simulink model "momentum_envelope_test"  (R2018b)
settings: Solver=ode4  StartTime=0.0  StopTime=500.0  FixedStep=0.1  MaxStep=1e-1  RelTol=1e-5  AbsTol=1e-5
undefined symbols (not defined in the file): DiscIntNeverNeededParam, fswParams
libraries: rwa_allocation_lib x1
settings Model: Creator=taylorreynolds  LastModifiedBy=taylorreynolds

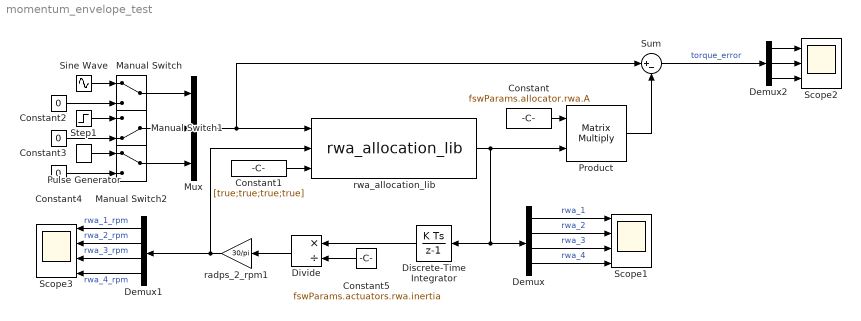
== system momentum_envelope_test ==
  Constant : Constant  Value=fswParams.allocator.rwa.A
  Constant1 : Constant  Value=[true;true;true;true]
  Constant2 : Constant  Value=0
  Constant3 : Constant  Value=0
  Constant4 : Constant  Value=0
  Constant5 : Constant  Value=fswParams.actuators.rwa.inertia
  Demux : Demux
  Demux1 : Demux
  Demux2 : Demux  Outputs=3
  Discrete-Time Integrator : DiscreteIntegrator  SampleTime=-1  ICPrevOutput=DiscIntNeverNeededParam  ICPrevScaledInput=DiscIntNeverNeededParam
  Divide : Product  Inputs=*/
  Manual Switch : ManualSwitch
  Manual Switch1 : ManualSwitch  CurrentSetting=0
  Manual Switch2 : ManualSwitch
  Mux : Mux  Inputs=3
  Product : Product  Multiplication=Matrix(*)
  Pulse Generator : DiscretePulseGenerator  PulseType=Time based  Amplitude=1e-3  Period=60  PulseWidth=5
  Scope1 : Scope  NumInputPorts=4
  Scope2 : Scope  NumInputPorts=3
  Scope3 : Scope  NumInputPorts=4
  Sine Wave : Sin  Amplitude=1e-4  Frequency=0.1  SampleTime=0
  Step1 : Step  After=1e-4  SampleTime=0
  Sum : Sum  Inputs=|+-
  radps_2_rpm1 : Gain  Gain=30/pi
  rwa_allocation_lib : rwa_allocation_lib/rwa_allocation_lib  SystemSampleTime=-1
  wires:
  Discrete-Time Integrator/1 -> Divide/1
  Mux/1 -> rwa_allocation_lib/1, Sum/1
  Manual Switch/1 -> Mux/1
  Manual Switch1/1 -> Mux/2
  Manual Switch2/1 -> Mux/3
  rwa_allocation_lib/1 -> Discrete-Time Integrator/1, Demux/1, Product/2
  Demux/1 -> Scope1/1  "rwa_1"
  Demux/2 -> Scope1/2  "rwa_2"
  Demux/3 -> Scope1/3  "rwa_3"
  Demux/4 -> Scope1/4  "rwa_4"
  Demux1/1 -> Scope3/1  "rwa_1_rpm"
  Demux1/2 -> Scope3/2  "rwa_2_rpm"
  Demux1/3 -> Scope3/3  "rwa_3_rpm"
  Demux1/4 -> Scope3/4  "rwa_4_rpm"
  radps_2_rpm1/1 -> rwa_allocation_lib/2, Demux1/1
  Constant/1 -> Product/1
  Product/1 -> Sum/2
  Demux2/1 -> Scope2/1
  Demux2/2 -> Scope2/2
  Demux2/3 -> Scope2/3
  Constant1/1 -> rwa_allocation_lib/3
  Sum/1 -> Demux2/1  "torque_error"
  Sine Wave/1 -> Manual Switch/1
  Constant2/1 -> Manual Switch/2
  Pulse Generator/1 -> Manual Switch2/1
  Constant3/1 -> Manual Switch1/2
  Step1/1 -> Manual Switch1/1
  Constant4/1 -> Manual Switch2/2
  Divide/1 -> radps_2_rpm1/1
  Constant5/1 -> Divide/2
